simulink model "dist_isol_tank"  (R2021b)
settings: Solver=VariableStepAuto  StartTime=0.0  StopTime=1000  RelTol=1e-3
libraries: dspsrcs4 x1
settings Model: Creator=billtubbs  LastModifiedBy=billtubbs

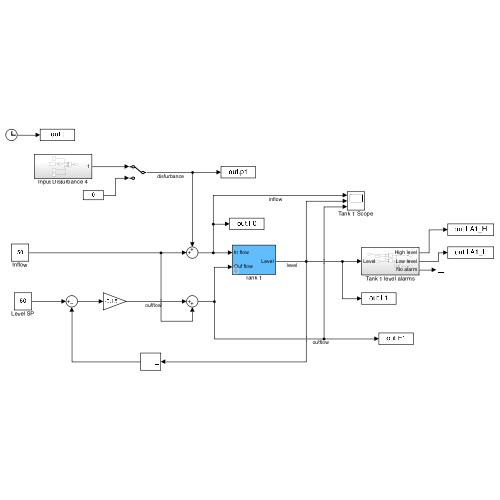
[thumbnail: Simulink's stored preview of the top-level diagram]
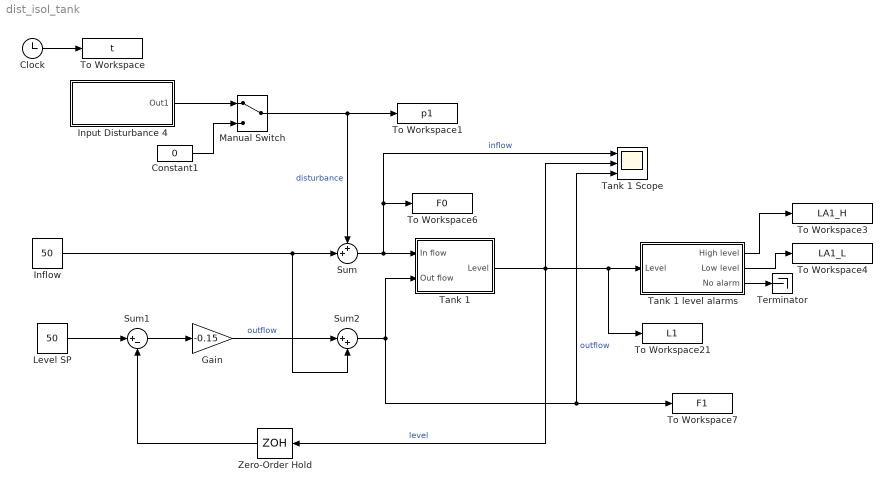
== system dist_isol_tank ==
  Clock : Clock
  Constant1 : Constant  Value=0  SampleTime=1
  Gain : Gain  Gain=-0.15
  Inflow : Constant  Value=50
  Input Disturbance 4 : Subsystem
  Level SP : Constant  Value=50
  Manual Switch : ManualSwitch
  Sum : Sum  Inputs=++|
  Sum1 : Sum  Inputs=|+-
  Sum2 : Sum  Inputs=|++
  Tank 1 : Subsystem  mask{K=0.05, y0=50}
  Tank 1 Scope : Scope  NumInputPorts=3
  Tank 1 level alarms : Subsystem
  Terminator : Terminator
  To Workspace : ToWorkspace  VariableName=t  SampleTime=1
  To Workspace1 : ToWorkspace  VariableName=p1  SampleTime=1
      settings: Save2DSignal=2-D array (concatenate along first dimension)
  To Workspace21 : ToWorkspace  VariableName=L1  SampleTime=1
  To Workspace3 : ToWorkspace  VariableName=LA1_H  SampleTime=1
  To Workspace4 : ToWorkspace  VariableName=LA1_L  SampleTime=1
  To Workspace6 : ToWorkspace  VariableName=F0  SampleTime=1
  To Workspace7 : ToWorkspace  VariableName=F1  SampleTime=1
  Zero-Order Hold : ZeroOrderHold  SampleTime=100
  wires:
  Clock/1 -> To Workspace/1
  Sum/1 -> Tank 1/1(In flow), Tank 1 Scope/1, To Workspace6/1  "inflow"
  Manual Switch/1 -> To Workspace1/1, Sum/1  "disturbance"
  Constant1/1 -> Manual Switch/2
  Input Disturbance 4/1(Out1) -> Manual Switch/1
  Inflow/1 -> Sum2/2, Sum/2
  Sum2/1 -> Tank 1 Scope/3, To Workspace7/1, Tank 1/2(Out flow)  "outflow"
  Tank 1 level alarms/3(No alarm) -> Terminator/1
  Tank 1 level alarms/2(Low level) -> To Workspace4/1
  Tank 1/1(Level) -> Zero-Order Hold/1, To Workspace21/1, Tank 1 level alarms/1(Level), Tank 1 Scope/2  "level"
  Tank 1 level alarms/1(High level) -> To Workspace3/1
  Level SP/1 -> Sum1/1
  Zero-Order Hold/1 -> Sum1/2
  Sum1/1 -> Gain/1
  Gain/1 -> Sum2/1  "outflow"

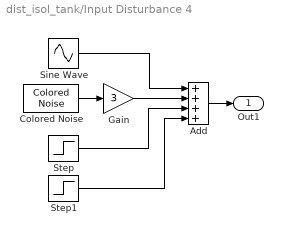
== system dist_isol_tank/Input Disturbance 4 ==
  Add : Sum  Inputs=++++
  Colored Noise : dspsrcs4/Colored Noise  Color=pink  InverseFrequencyPower=1  BoundedOutput=off  NumChannels=1  OutputDataType=double  SamplesPerFrame=1  SampleTime=1  RandomStream=mt19937ar with seed  Seed=67  SimulateUsing=Interpreted execution
      settings: SourceProductBaseCode=DS
  Gain : Gain  Gain=3
  Sine Wave : Sin  Amplitude=0  Frequency=1/60  SampleTime=0
  Step : Step  Time=100  After=0  SampleTime=0
  Step1 : Step  Time=200  After=0  SampleTime=0
  Out1 : Outport
  wires:
  Colored Noise/1 -> Gain/1
  Gain/1 -> Add/2
  Step/1 -> Add/3
  Sine Wave/1 -> Add/1
  Add/1 -> Out1/1
  Step1/1 -> Add/4

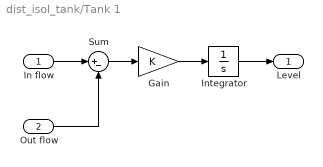
== system dist_isol_tank/Tank 1 ==
  In flow : Inport
  Out flow : Inport  Port=2
  Gain : Gain  Gain=K
  Integrator : Integrator  InitialCondition=y0
  Sum : Sum  Inputs=|+-
  Level : Outport  InitialOutput=0
  wires:
  Sum/1 -> Gain/1
  Integrator/1 -> Level/1
  In flow/1 -> Sum/1
  Out flow/1 -> Sum/2
  Gain/1 -> Integrator/1

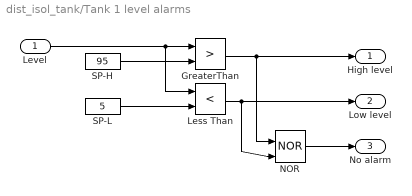
== system dist_isol_tank/Tank 1 level alarms ==
  Level : Inport
  GreaterThan : RelationalOperator  Operator=>  OutDataTypeStr=boolean  RndMeth=Simplest
  Less Than : RelationalOperator  Operator=<  OutDataTypeStr=boolean  RndMeth=Simplest
  NOR : Logic  Operator=NOR  IconShape=distinctive  AllPortsSameDT=off  OutDataTypeStr=boolean
  SP-H : Constant  Value=95
  SP-L : Constant  Value=5
  High level : Outport
  Low level : Outport  Port=2
  No alarm : Outport  Port=3
  wires:
  Level/1 -> Less Than/1, GreaterThan/1
  SP-L/1 -> Less Than/2
  GreaterThan/1 -> High level/1, NOR/1
  SP-H/1 -> GreaterThan/2
  Less Than/1 -> NOR/2, Low level/1
  NOR/1 -> No alarm/1
